simulink model "gain_calculation_sim"  (R2020b)
settings: Solver=FixedStepAuto  StartTime=0.0  StopTime=simulation_time  RelTol=1e-3
InitFcn:
  | initCallback
StopFcn:
  | stopCallback
values from neighbouring files (symbols this model uses):
  fs = audio_fs * fft_up_sample_rate    (= 6144000)    [modelparameters.m]
settings Model: Creator=t96f346  LastModifiedBy=conno
settings DataIOCC: ReturnWorkspaceOutputs=off

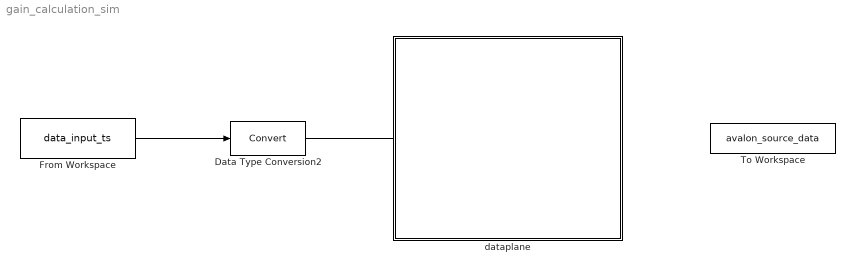
== system gain_calculation_sim ==
  Data Type Conversion2 : DataTypeConversion  RndMeth=Nearest  SaturateOnIntegerOverflow=on
  From Workspace : FromWorkspace  VariableName=data_input_ts  SampleTime=1/fs
  To Workspace : ToWorkspace  VariableName=avalon_source_data  SampleTime=-1
  dataplane : Subsystem  TreatAsAtomicUnit=on
  wires:
  From Workspace/1 -> Data Type Conversion2/1
  Data Type Conversion2/1 -> ?
  ? -> To Workspace/1

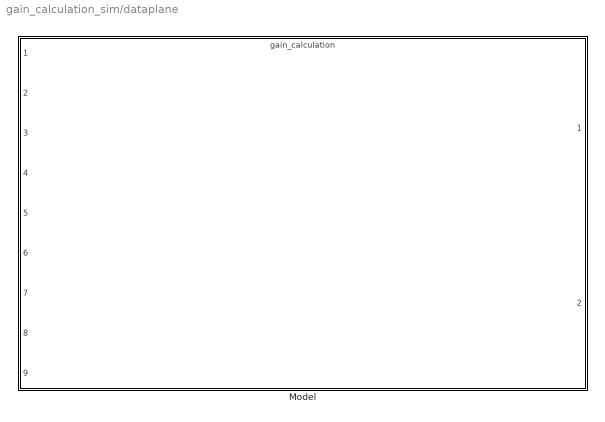
== system gain_calculation_sim/dataplane ==
  Model : ModelReference  ModelNameDialog=gain_calculation.slx  SimulationMode=Normal  ModelReferenceVersion=1.8
